simulink model "quadrotorsim_Equations_New_V6B_RC_Only"  (R2019a)
settings: Solver=FixedStepAuto  StartTime=0.0  StopTime=10  FixedStep=1  RelTol=1e-3  EnableMultiTasking=on
undefined symbols (not defined in the file): dev, Main, pwm_output0, px4
libraries: simulink x2, px4lib x1
settings Model: ExtModeTrigDuration=10  Creator=samirbo  LastModifiedBy=MEDELEON
settings SolverCC: PositivePriorityOrder=on
settings DataIOCC: LimitDataPoints=on  SaveFormat=Array  ReturnWorkspaceOutputs=off
settings OptimizationCC: EnhancedBackFolding=on  PassReuseOutputArgsAs=Individual arguments  ExpressionDepthLimit=2147483647  InitFltsAndDblsToZero=on  MaxStackSize=64  OptimizeBlockOrder=speed  DifferentSizesBufferReuse=on  OptimizationCustomize=off
settings DebuggingCC: SaveWithParameterizedLinksMsg=none  UnderspecifiedInitializationDetection=Classic  MergeDetectMultiDrivingBlocksExec=none  SignalResolutionControl=TryResolveAllWithWarning  SolverPrmCheckMsg=warning  MultiTaskDSMMsg=warning  MultiTaskCondExecSysMsg=none  ParameterPrecisionLossMsg=none  ParameterTunabilityLossMsg=error  FcnCallInpInsideContextMsg=warning  StateNameClashWarn=warning  SFUnexpectedBacktrackingDiag=warning  SFNoUnconditionalDefaultTransitionDiag=warning  SFExecutionAtInitializationDiag=none  ArithmeticOperatorsInVariantConditions=warning
settings HardwareCC: ProdBitPerPointer=32  ProdBitPerSizeT=32  ProdBitPerPtrDiffT=32  ProdLargestAtomicInteger=Long  ProdLargestAtomicFloat=Double  ProdWordSize=32  ProdLongLongMode=on  ProdHWDeviceType=ARM Compatible->ARM Cortex
settings ModelReferenceCC: PropagateSignalLabelsOutOfModel=off
settings SFSimCC: SimUseLocalCustomCode=off  MATLABDynamicMemAlloc=off
settings RTWCC: SystemTargetFile=ert.tlc  HardwareBoard=PX4 Pixhawk 2.1 (Cube)  TLCOptions="-aInlineSetEventsForThisBaseRateFcn=TLC_FALSE -aSuppressMultiTaskScheduler=TLC_FALSE  -aRateBasedStepFcn=0"  TemplateMakefile=ert_default_tmf  GenerateReport=on  RTWUseLocalCustomCode=off  Toolchain=GNU Tools for PX4 Autopilots  IncludeHyperlinkInReport=on  LaunchReport=on  TargetLang=C++  GenerateTraceInfo=on  GenerateTraceReport=on  GenerateTraceReportSl=on  GenerateTraceReportSf=on  GenerateTraceReportEml=on  CheckMdlBeforeBuild=Error
settings CodeAppCC: ForceParamTrailComments=on  IgnoreCustomStorageClasses=off  OperatorAnnotations=on  SimulinkDataObjDesc=on  SFDataObjDesc=on  InsertBlockDesc=on
settings ConfigComp: CovMetricSettings=dw  CovHtmlReporting=on  CovSaveCumulativeToWorkspaceVar=on  CovSaveSingleToWorkspaceVar=on  CovExternalEMLEnable=off

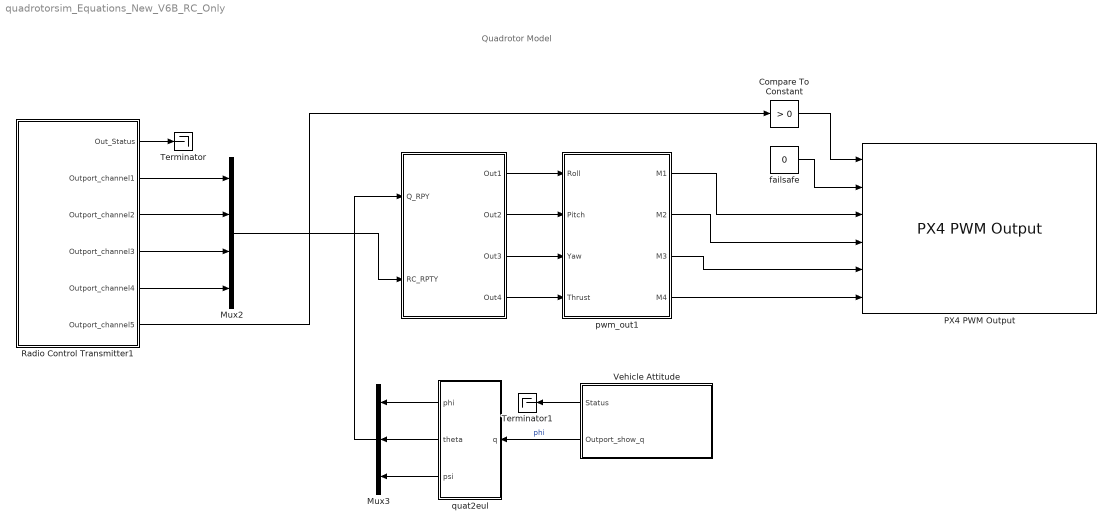
== system quadrotorsim_Equations_New_V6B_RC_Only ==
  note: Quadrotor Model
  " " : Subsystem
      mask Display: disp('Control System')
  Compare To Constant : simulink/Logic and Bit Operations/Compare To Constant  relop=>  const=0  OutDataTypeStr=boolean
  Mux2 : Mux
  Mux3 : Mux  Inputs=3
  PX4 PWM Output : px4lib/PX4 PWM Output  pwmDevice=Main (/dev/pwm_output0)  pwmChannel1_=on  pwmChannel2_=on  pwmChannel3_=on  pwmChannel4_=on  pwmChannel5_=off  pwmChannel6_=off  pwmChannel7_=off  pwmChannel8_=off  forceTerminateFailsafe=off  outputErrorStatus=off
      settings: SourceProductName=Embedded Coder Support Package for PX4 Autopilots  SourceProductBaseCode=PX4AUTOPILOTS
  Radio Control Transmitter1 : Subsystem  AncestorBlock=px4Sensorslib/Radio Control Transmitter  mask(PX4 Radio Control Transmitter){channel1=on, channel2=on, channel3=on, channel4=on, channel5=on, channel6=off, channel7=off, channel8=off, channel_count=off, rssi=off, rc_input_source=off, timestamp_last_signal=off, time_stamp=off, sampleTime=-1, BlockingMode=off, BlockTimeout=5}
      mask prompts: channel1 "px4:blockmask:uORBRCBlockMaskCh1"; channel2 "px4:blockmask:uORBRCBlockMaskCh2"; channel3 "px4:blockmask:uORBRCBlockMaskCh3"; channel4 "px4:blockmask:uORBRCBlockMaskCh4"; channel5 "px4:blockmask:uORBRCBlockMaskCh5"; channel6 "px4:blockmask:uORBRCBlockMaskCh6"; channel7 "px4:blockmask:uORBRCBlockMaskCh7"; channel8 "px4:blockmask:uORBRCBlockMaskCh8"; channel_count "px4:blockmask:uORBRCBlockMaskChCount"; rssi "px4:blockmask:uORBRCBlockMaskRSSI"; rc_input_source "px4:blockmask:uORBRCBlockMaskRCSource"; timestamp_last_signal "px4:blockmask:uORBRCBlockMaskRCTimestampLastSignal"; time_stamp "px4:blockmask:uORBRCBlockMaskTs"; sampleTime "px4:blockmask:SampleTimePrompt"; BlockingMode "px4:blockmask:SubscriberBlockingMode"; BlockTimeout "px4:blockmask:SubscriberBlockingModeTimeout"
      mask help: px4:blockmask:uORBRCBlockMaskDescription
      mask init:
      | signal_names = {'channel_1','channel_2','channel_3','channel_4',...
      |                         'channel_5','channel_6','channel_7','channel_8',...
      |                         '<channel_count>','<rssi>',...
      |                         '<input_source>','<timestamp_last_signal>','<timestamp>'};
      | output_port_names = {'Ch 1','Ch 2','Ch 3',...
      |                         'Ch 4','Ch 5','Ch 6','Ch 7',...
      |                         'Ch 8','Num Ch','RSSI',...
      |                         'RC Source','Last valid time','Timestamp'...
      |                         };
      | mask_image = 'mask_input_rc.png';                    
      | imfilename = fullfile(codertarget.pixhawk.internal.getSpPkgRootDir, 'resources', mask_image);
      | px4.internal.block.CommonuORBTopicMask.commonMaskCallback(gcb,signal_names,output_port_names,imfilename);
      mask Help: eval('codertarget.internal.helpView(''px4'',''px4librctransmitter'')');
      mask TypeOptions sampleTime: PX4 uORB Read/sampleTime
      mask TypeOptions BlockingMode: PX4 uORB Read/BlockingMode
      mask Callback BlockingMode: px4.internal.block.CommonuORBTopicMask.blockingModeCallback(gcb);
      mask TypeOptions BlockTimeout: PX4 uORB Read/BlockTimeout
      mask DialogControl Container10 Prompt: px4:blockmask:uORBRCBlockMainTab
      mask DialogControl Container14 Prompt: px4:blockmask:uORBRCBlockChSelection
      mask DialogControl Container17 Prompt: px4:blockmask:uORBRCBlockAdditionalOp
      mask DialogControl Container19 Prompt: px4:blockmask:uORBRCBlockAdvancedTab
      mask Display:
      | color('white');
      | plot([100,100,100,100],[100,100,100,100]);
      | plot([0,0,0,0],[0,0,0,0]);
      | image('C:\ProgramData\MATLAB\SupportPackages\R2018b\toolbox\target\supportpackages\px4\resources\mask_input_rc.png','center')
      | color('blue');
      | text(0.25, 0.9, 'PX4', 'horizontalAlignment', 'right');
      | color('black');
      | port_label('output',1,'Status');
      | port_label('output',2,'Ch 1');
      | port_label('output',3,'Ch 2');
      | port_label('output',4,'Ch 3');
      | port_label('output',5,'Ch 4');
      | port_label('output',6,'Ch 5');
  Terminator : Terminator
  Terminator1 : Terminator
  Vehicle Attitude : Subsystem  AncestorBlock=px4Sensorslib/Vehicle Attitude  mask(PX4 Vehicle Attitude){rollRate=off, pitchRate=off, yawRate=off, quaternion=on, uorbTimeStamp=off, BlockingMode=off, BlockTimeout=0.001, sampleTime=-1}
      mask prompts: rollRate "Roll Rate"; pitchRate "Pitch Rate"; yawRate "Yaw Rate"; quaternion "Quaternion (NED)"; uorbTimeStamp "Timestamp"; BlockingMode "px4:blockmask:SubscriberBlockingMode"; BlockTimeout "px4:blockmask:SubscriberBlockingModeTimeout"; sampleTime "px4:blockmask:SampleTimePrompt"
      mask help: px4:blockmask:VehicleAttitueBlockMaskDescription
      mask init:
      | signal_names = {'<rollspeed>','<pitchspeed>','<yawspeed>',...
      |     '<q>','<timestamp>'};
      | output_port_names = {'Roll rate','Pitch rate',...
      |     'Yaw rate','Quaternion','Timestamp'};
      | mask_image = fullfile(codertarget.pixhawk.internal.getSpPkgRootDir,...
      |     'resources','mask_vehicle_attitude.png');
      | 
      | px4.internal.block.CommonuORBTopicMask.commonMaskCallback(gcb,...
      |     signal_names,output_port_names,mask_image);
      mask Help: eval('codertarget.internal.helpView(''px4'' ,''px4libvehicleattitude'')')
      mask TypeOptions BlockingMode: PX4 uORB Read/BlockingMode
      mask Callback BlockingMode: px4.internal.block.CommonuORBTopicMask.blockingModeCallback(gcb);
      mask TypeOptions BlockTimeout: PX4 uORB Read/BlockTimeout
      mask TypeOptions sampleTime: PX4 uORB Read/sampleTime
      mask DialogControl Container6 Prompt: Main
      mask DialogControl Container8 Prompt: Advanced
      mask Display:
      | color('white');
      | plot([100,100,100,100],[100,100,100,100]);
      | plot([0,0,0,0],[0,0,0,0]);
      | image('C:\ProgramData\MATLAB\SupportPackages\R2018b\toolbox\target\supportpackages\px4\resources\mask_vehicle_attitude.png','center')
      | color('blue');
      | text(0.25, 0.9, 'PX4', 'horizontalAlignment', 'right');
      | color('black');
      | port_label('output',1,'Status');
      | port_label('output',2,'Quaternion');
  failsafe : Constant  Value=0  OutDataTypeStr=boolean  SampleTime=-1
  pwm_out1 : MATLAB Function  TreatAsAtomicUnit=on
  quat2eul : MATLAB Function  TreatAsAtomicUnit=on
  wires:
  Radio Control Transmitter1/2(Outport_channel1) -> Mux2/1
  Radio Control Transmitter1/3(Outport_channel2) -> Mux2/2
  Radio Control Transmitter1/4(Outport_channel3) -> Mux2/3
  Radio Control Transmitter1/5(Outport_channel4) -> Mux2/4
  quat2eul/2(theta) -> Mux3/2
  quat2eul/1(phi) -> Mux3/1
  quat2eul/3(psi) -> Mux3/3
  Vehicle Attitude/2(Outport_show_q) -> quat2eul/1(q)  "phi"
  " "/1(Out1) -> pwm_out1/1(Roll)
  " "/2(Out2) -> pwm_out1/2(Pitch)
  " "/3(Out3) -> pwm_out1/3(Yaw)
  " "/4(Out4) -> pwm_out1/4(Thrust)
  pwm_out1/1(M1) -> PX4 PWM Output/3
  pwm_out1/2(M2) -> PX4 PWM Output/4
  pwm_out1/3(M3) -> PX4 PWM Output/5
  pwm_out1/4(M4) -> PX4 PWM Output/6
  Mux3/1 -> " "/1(Q_RPY)
  Mux2/1 -> " "/2(RC_RPTY)
  Radio Control Transmitter1/1(Out_Status) -> Terminator/1
  Vehicle Attitude/1(Status) -> Terminator1/1
  Radio Control Transmitter1/6(Outport_channel5) -> Compare To Constant/1
  failsafe/1 -> PX4 PWM Output/2
  Compare To Constant/1 -> PX4 PWM Output/1

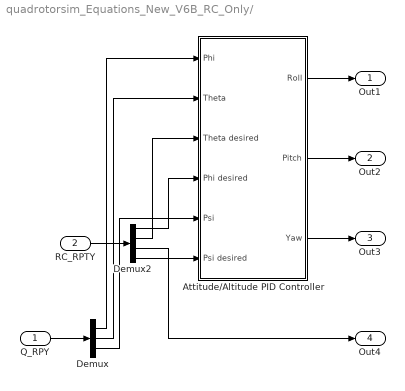
== system quadrotorsim_Equations_New_V6B_RC_Only/  ==
  Q_RPY : Inport
  RC_RPTY : Inport  Port=2
  Attitude/Altitude PID Controller : Subsystem
  Demux : Demux  Outputs=3
  Demux2 : Demux
  Out1 : Outport
  Out2 : Outport  Port=2
  Out3 : Outport  Port=3
  Out4 : Outport  Port=4
  wires:
  Q_RPY/1 -> Demux/1
  Demux/1 -> Attitude/Altitude PID Controller/1(Phi)
  Demux/2 -> Attitude/Altitude PID Controller/2(Theta)
  Demux/3 -> Attitude/Altitude PID Controller/5(Psi)
  RC_RPTY/1 -> Demux2/1
  Attitude/Altitude PID Controller/1(Roll) -> Out1/1
  Attitude/Altitude PID Controller/2(Pitch) -> Out2/1
  Attitude/Altitude PID Controller/3(Yaw) -> Out3/1
  Demux2/1 -> Attitude/Altitude PID Controller/4(Phi desired)
  Demux2/2 -> Attitude/Altitude PID Controller/3(Theta desired)
  Demux2/4 -> Attitude/Altitude PID Controller/6(Psi desired)
  Demux2/3 -> Out4/1

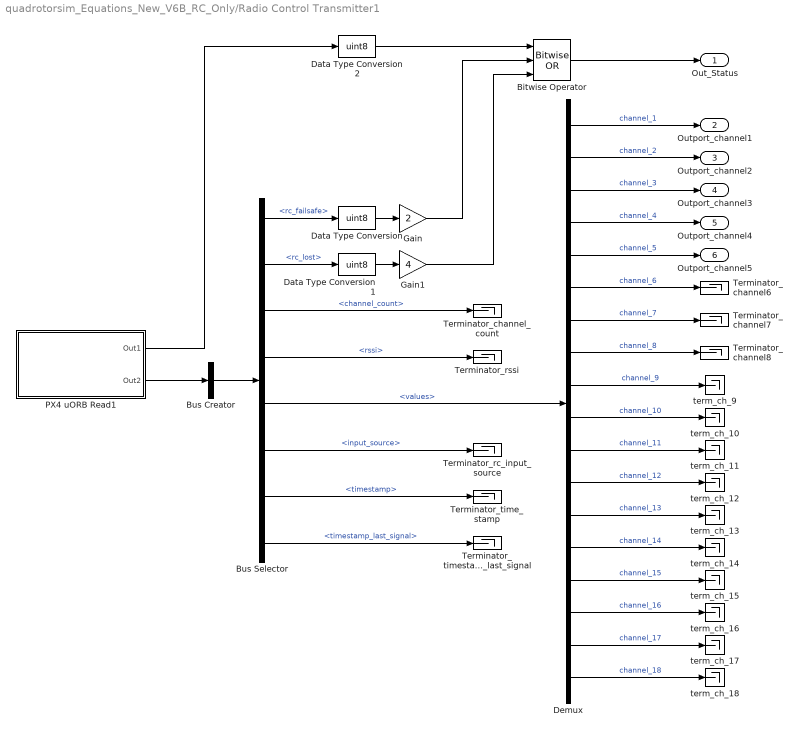
== system quadrotorsim_Equations_New_V6B_RC_Only/Radio Control Transmitter1 ==
  Bitwise Operator : simulink/Logic and Bit Operations/Bitwise Operator  logicop=OR  UseBitMask=off  NumInputPorts=3  BitMask=bin2dec('11011001')  BitMaskRealWorld=Stored Integer
  Bus Creator : BusCreator  Inputs=1
  Bus Selector : BusSelector  OutputSignals=rc_failsafe,rc_lost,channel_count,rssi,values,input_source,timestamp,timestamp_last_signal
  Data Type Conversion : DataTypeConversion  OutDataTypeStr=uint8
  Data Type Conversion1 : DataTypeConversion  OutDataTypeStr=uint8
  Data Type Conversion2 : DataTypeConversion  OutDataTypeStr=uint8
  Demux : Demux  Outputs=18
  Gain : Gain  Gain=2  OutDataTypeStr=uint8
  Gain1 : Gain  Gain=4  OutDataTypeStr=uint8
  PX4 uORB Read1 : Subsystem  AncestorBlock=px4uORBlib/PX4 uORB Read  mask(PX4 uORB Read){uORBTopic=input_rc, sampleTime=-1, BlockingMode=off, BlockTimeout=1e-3}
      mask prompts: uORBTopic "px4:blockmask:TopicPrompt"; sampleTime "px4:blockmask:SampleTimePrompt"; BlockingMode "px4:blockmask:SubscriberBlockingMode"; BlockTimeout "px4:blockmask:SubscriberBlockingModeTimeout"
      mask help: px4:blockmask:SubscriberBlockMaskDescription
      mask init:
      | px4.internal.block.SubscribeBlockMask.dispatch('maskInitialize', gcb);
      settings: ModelCloseFcn=px4.internal.block.SubscribeBlockMask.dispatch('modelCloseFcn', gcb);
      mask Help: eval('codertarget.internal.helpView(''px4'',''px4libuorbread'')');
      mask TypeOptions uORBTopic: SourceBlock/uORBTopic
      mask Callback uORBTopic: px4.internal.block.SubscribeBlockMask.dispatch('topicEdit', gcb);
      mask TypeOptions sampleTime: SourceBlock/SampleTime
      mask TypeOptions BlockingMode: SourceBlock/BlockingMode
      mask Callback BlockingMode: px4.internal.block.SubscribeBlockMask.dispatch('blockingModeSelect', gcb);
      mask TypeOptions BlockTimeout: SourceBlock/BlockTimeout
      mask DialogControl ContainerMain Prompt: px4:blockmask:MainTabTitle
      mask DialogControl topicSelectButton Prompt: px4:blockmask:SelectPrompt
      mask DialogControl topicSelectButton Callback: px4.internal.block.SubscribeBlockMask.dispatch('topicSelect', gcb);
      mask DialogControl ContainerAdvanced Prompt: px4:blockmask:AdvancedTabTitle
      mask Display:
      | color('blue');
      | text(0.2, 0.90, 'PX4', 'horizontalAlignment', 'right');
      | color('black');
      | text(0.5, 0.60, 'uORB Read', 'horizontalAlignment', 'center');
      | if length(uORBTopic) > 16
      |   text(0.83, 0.15, uORBTopic, 'horizontalAlignment', 'right');
      | else
      |   text(0.5, 0.15, uORBTopic, 'horizontalAlignment', 'center');
      | end
      | port_label('output', 1, 'Status');
      | port_label('output', 2, 'Msg');
  Terminator_channel6 : Terminator
  Terminator_channel7 : Terminator
  Terminator_channel8 : Terminator
  Terminator_channel_count : Terminator
  Terminator_rc_input_source : Terminator
  Terminator_rssi : Terminator
  Terminator_time_stamp : Terminator
  Terminator_timestamp_last_signal : Terminator
  "term_ch_10 " : Terminator
  term_ch_{9,11..18} (9 alike) : Terminator
  Out_Status : Outport
  Outport_channel1 : Outport  Port=2
  Outport_channel2 : Outport  Port=3
  Outport_channel3 : Outport  Port=4
  Outport_channel4 : Outport  Port=5
  Outport_channel5 : Outport  Port=6
  wires:
  Data Type Conversion2/1 -> Bitwise Operator/1
  Gain1/1 -> Bitwise Operator/3
  Gain/1 -> Bitwise Operator/2
  PX4 uORB Read1/1(Out1) -> Data Type Conversion2/1
  Bitwise Operator/1 -> Out_Status/1
  Data Type Conversion1/1 -> Gain1/1
  Data Type Conversion/1 -> Gain/1
  Bus Selector/8 -> Terminator_timestamp_last_signal/1  "<timestamp_last_signal>"
  Demux/11 -> term_ch_11/1  "channel_11"
  Demux/3 -> Outport_channel3/1  "channel_3"
  Demux/16 -> term_ch_16/1  "channel_16"
  Demux/13 -> term_ch_13/1  "channel_13"
  Demux/18 -> term_ch_18/1  "channel_18"
  Demux/15 -> term_ch_15/1  "channel_15"
  Bus Selector/3 -> Terminator_channel_count/1  "<channel_count>"
  Demux/17 -> term_ch_17/1  "channel_17"
  Demux/9 -> term_ch_9/1  "channel_9"
  Bus Selector/5 -> Demux/1  "<values>"
  Bus Selector/6 -> Terminator_rc_input_source/1  "<input_source>"
  Demux/10 -> "term_ch_10 "/1  "channel_10"
  Demux/1 -> Outport_channel1/1  "channel_1"
  Demux/12 -> term_ch_12/1  "channel_12"
  Demux/14 -> term_ch_14/1  "channel_14"
  Demux/6 -> Terminator_channel6/1  "channel_6"
  Demux/5 -> Outport_channel5/1  "channel_5"
  Demux/7 -> Terminator_channel7/1  "channel_7"
  Demux/2 -> Outport_channel2/1  "channel_2"
  Demux/8 -> Terminator_channel8/1  "channel_8"
  Demux/4 -> Outport_channel4/1  "channel_4"
  Bus Selector/4 -> Terminator_rssi/1  "<rssi>"
  Bus Selector/1 -> Data Type Conversion/1  "<rc_failsafe>"
  Bus Selector/2 -> Data Type Conversion1/1  "<rc_lost>"
  Bus Selector/7 -> Terminator_time_stamp/1  "<timestamp>"
  PX4 uORB Read1/2(Out2) -> Bus Creator/1
  Bus Creator/1 -> Bus Selector/1

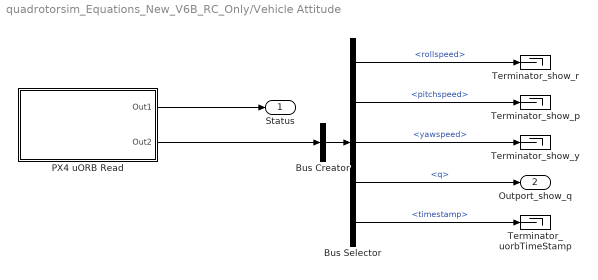
== system quadrotorsim_Equations_New_V6B_RC_Only/Vehicle Attitude ==
  Bus Creator : BusCreator  Inputs=1
  Bus Selector : BusSelector  OutputSignals=rollspeed,pitchspeed,yawspeed,q,timestamp
  PX4 uORB Read : Subsystem  AncestorBlock=px4uORBlib/PX4 uORB Read  mask(PX4 uORB Read){uORBTopic=vehicle_attitude, sampleTime=-1, BlockingMode=off, BlockTimeout=0.001}
      mask prompts: uORBTopic "px4:blockmask:TopicPrompt"; sampleTime "px4:blockmask:SampleTimePrompt"; BlockingMode "px4:blockmask:SubscriberBlockingMode"; BlockTimeout "px4:blockmask:SubscriberBlockingModeTimeout"
      mask help: px4:blockmask:SubscriberBlockMaskDescription
      mask init:
      | px4.internal.block.SubscribeBlockMask.dispatch('maskInitialize', gcb);
      settings: ModelCloseFcn=px4.internal.block.SubscribeBlockMask.dispatch('modelCloseFcn', gcb);
      mask Help: eval('codertarget.internal.helpView(''px4'',''px4libuorbread'')');
      mask TypeOptions uORBTopic: SourceBlock/uORBTopic
      mask Callback uORBTopic: px4.internal.block.SubscribeBlockMask.dispatch('topicEdit', gcb);
      mask TypeOptions sampleTime: SourceBlock/SampleTime
      mask TypeOptions BlockingMode: SourceBlock/BlockingMode
      mask Callback BlockingMode: px4.internal.block.SubscribeBlockMask.dispatch('blockingModeSelect', gcb);
      mask TypeOptions BlockTimeout: SourceBlock/BlockTimeout
      mask DialogControl ContainerMain Prompt: px4:blockmask:MainTabTitle
      mask DialogControl topicSelectButton Prompt: px4:blockmask:SelectPrompt
      mask DialogControl topicSelectButton Callback: px4.internal.block.SubscribeBlockMask.dispatch('topicSelect', gcb);
      mask DialogControl ContainerAdvanced Prompt: px4:blockmask:AdvancedTabTitle
      mask Display:
      | color('blue');
      | text(0.2, 0.90, 'PX4', 'horizontalAlignment', 'right');
      | color('black');
      | text(0.5, 0.60, 'uORB Read', 'horizontalAlignment', 'center');
      | if length(uORBTopic) > 16
      |   text(0.83, 0.15, uORBTopic, 'horizontalAlignment', 'right');
      | else
      |   text(0.5, 0.15, uORBTopic, 'horizontalAlignment', 'center');
      | end
      | port_label('output', 1, 'Status');
      | port_label('output', 2, 'Msg');
  Terminator_show_p : Terminator
  Terminator_show_r : Terminator
  Terminator_show_y : Terminator
  Terminator_uorbTimeStamp : Terminator
  Status : Outport
  Outport_show_q : Outport  Port=2
  wires:
  Bus Selector/5 -> Terminator_uorbTimeStamp/1  "<timestamp>"
  Bus Selector/4 -> Outport_show_q/1  "<q>"
  Bus Selector/1 -> Terminator_show_r/1  "<rollspeed>"
  PX4 uORB Read/1(Out1) -> Status/1
  Bus Selector/2 -> Terminator_show_p/1  "<pitchspeed>"
  Bus Selector/3 -> Terminator_show_y/1  "<yawspeed>"
  PX4 uORB Read/2(Out2) -> Bus Creator/1
  Bus Creator/1 -> Bus Selector/1

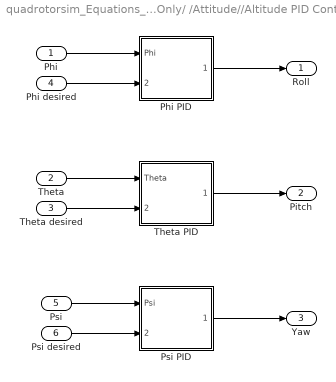
== system quadrotorsim_Equations_New_V6B_RC_Only/ /Attitude//Altitude PID Controller ==
  Phi : Inport
  Theta : Inport  Port=2
  Theta desired : Inport  Port=3
  Phi desired : Inport  Port=4
  Psi : Inport  Port=5
  Psi desired : Inport  Port=6
  Phi PID : Subsystem
  Psi PID : Subsystem
  Theta PID : Subsystem
  Roll : Outport
  Pitch : Outport  Port=2
  Yaw : Outport  Port=3
  wires:
  Phi desired/1 -> Phi PID/2(Phi desired)
  Phi/1 -> Phi PID/1(Phi)
  Psi desired/1 -> Psi PID/2(Psi desired)
  Psi/1 -> Psi PID/1(Psi)
  Theta desired/1 -> Theta PID/2(Theta desired)
  Theta/1 -> Theta PID/1(Theta)
  Phi PID/1(p desired) -> Roll/1
  Psi PID/1(r desired) -> Yaw/1
  Theta PID/1(q desired) -> Pitch/1

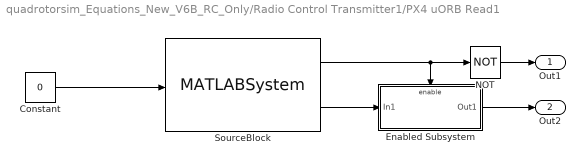
== system quadrotorsim_Equations_New_V6B_RC_Only/Radio Control Transmitter1/PX4 uORB Read1 ==
  Constant : Constant  Value=0  SampleTime=-1
  Enabled Subsystem : Subsystem  TreatAsAtomicUnit=on
  NOT : Logic  Operator=NOT  IconShape=distinctive  AllPortsSameDT=off  OutDataTypeStr=boolean
  SourceBlock : MATLABSystem  InitFcn=px4.internal.block.SubscribeBlockMask.dispatch('sysobjInitFcn', gcb);  System=px4.internal.block.Subscriber  uORBTopic=input_rc  SLBusName=px4_Bus_input_rc  SampleTime=-1  BlockingMode=off  BlockTimeout=1e-3
      mask Type: px4.internal.block.Subscriber
      mask Display:
      | disp('Subscriber');
      | port_label('input',1,'busstruct');
      | port_label('output',1,'isNewData');
      | port_label('output',2,'msg');
  Out1 : Outport
  Out2 : Outport  Port=2
  wires:
  NOT/1 -> Out1/1
  Enabled Subsystem/1(Out1) -> Out2/1
  SourceBlock/1 -> NOT/1, Enabled Subsystem/Enable
  SourceBlock/2 -> Enabled Subsystem/1(In1)
  Constant/1 -> SourceBlock/1

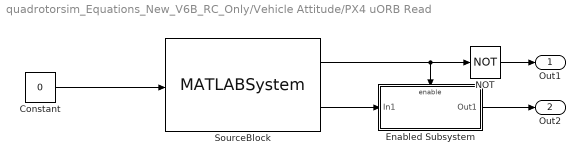
== system quadrotorsim_Equations_New_V6B_RC_Only/Vehicle Attitude/PX4 uORB Read ==
  Constant : Constant  Value=0  SampleTime=-1
  Enabled Subsystem : Subsystem  TreatAsAtomicUnit=on
  NOT : Logic  Operator=NOT  IconShape=distinctive  AllPortsSameDT=off  OutDataTypeStr=boolean
  SourceBlock : MATLABSystem  InitFcn=px4.internal.block.SubscribeBlockMask.dispatch('sysobjInitFcn', gcb);  System=px4.internal.block.Subscriber  uORBTopic=vehicle_attitude  SLBusName=px4_Bus_vehicle_attitude  SampleTime=-1  BlockingMode=off  BlockTimeout=0.001
      mask Type: px4.internal.block.Subscriber
      mask Display:
      | disp('Subscriber');
      | port_label('input',1,'busstruct');
      | port_label('output',1,'isNewData');
      | port_label('output',2,'msg');
  Out1 : Outport
  Out2 : Outport  Port=2
  wires:
  NOT/1 -> Out1/1
  Enabled Subsystem/1(Out1) -> Out2/1
  SourceBlock/1 -> NOT/1, Enabled Subsystem/Enable
  SourceBlock/2 -> Enabled Subsystem/1(In1)
  Constant/1 -> SourceBlock/1

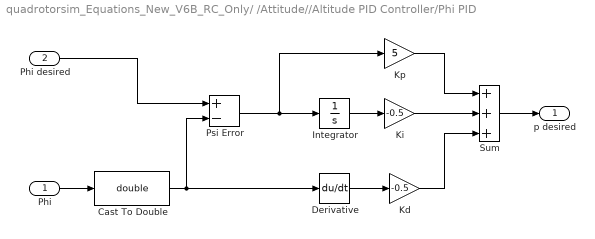
== system quadrotorsim_Equations_New_V6B_RC_Only/ /Attitude//Altitude PID Controller/Phi PID ==
  Phi : Inport
  Phi desired : Inport  Port=2
  Cast To Double : DataTypeConversion  OutDataTypeStr=double
  Derivative : Derivative
  Integrator : Integrator
  Kd : Gain  Gain=-0.5
  Ki : Gain  Gain=-0.5
  Kp : Gain  Gain=5
  Psi Error : Sum  Inputs=+-
  Sum : Sum  Inputs=+++
  p desired : Outport
  wires:
  Phi desired/1 -> Psi Error/1
  Derivative/1 -> Kd/1
  Kp/1 -> Sum/1
  Sum/1 -> p desired/1
  Psi Error/1 -> Integrator/1, Kp/1
  Integrator/1 -> Ki/1
  Kd/1 -> Sum/3
  Ki/1 -> Sum/2
  Phi/1 -> Cast To Double/1
  Cast To Double/1 -> Psi Error/2, Derivative/1

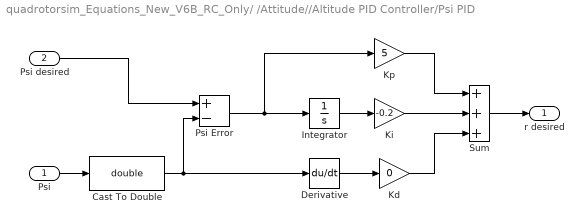
== system quadrotorsim_Equations_New_V6B_RC_Only/ /Attitude//Altitude PID Controller/Psi PID ==
  Psi : Inport
  Psi desired : Inport  Port=2
  Cast To Double : DataTypeConversion  OutDataTypeStr=double
  Derivative : Derivative
  Integrator : Integrator
  Kd : Gain  Gain=0
  Ki : Gain  Gain=-0.2
  Kp : Gain  Gain=5
  Psi Error : Sum  Inputs=+-
  Sum : Sum  Inputs=+++
  r desired : Outport
  wires:
  Psi desired/1 -> Psi Error/1
  Derivative/1 -> Kd/1
  Kp/1 -> Sum/1
  Sum/1 -> r desired/1
  Psi Error/1 -> Integrator/1, Kp/1
  Integrator/1 -> Ki/1
  Kd/1 -> Sum/3
  Ki/1 -> Sum/2
  Psi/1 -> Cast To Double/1
  Cast To Double/1 -> Psi Error/2, Derivative/1

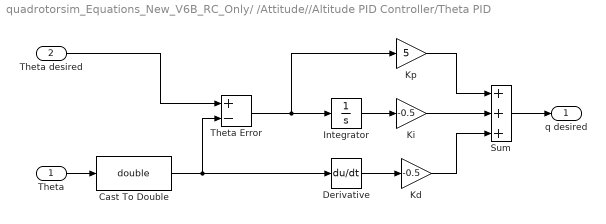
== system quadrotorsim_Equations_New_V6B_RC_Only/ /Attitude//Altitude PID Controller/Theta PID ==
  Theta : Inport
  Theta desired : Inport  Port=2
  Cast To Double : DataTypeConversion  OutDataTypeStr=double
  Derivative : Derivative
  Integrator : Integrator
  Kd : Gain  Gain=-0.5
  Ki : Gain  Gain=-0.5
  Kp : Gain  Gain=5
  Sum : Sum  Inputs=+++
  Theta Error : Sum  Inputs=+-
  q desired : Outport
  wires:
  Theta desired/1 -> Theta Error/1
  Derivative/1 -> Kd/1
  Kp/1 -> Sum/1
  Sum/1 -> q desired/1
  Theta Error/1 -> Integrator/1, Kp/1
  Integrator/1 -> Ki/1
  Kd/1 -> Sum/3
  Ki/1 -> Sum/2
  Theta/1 -> Cast To Double/1
  Cast To Double/1 -> Derivative/1, Theta Error/2

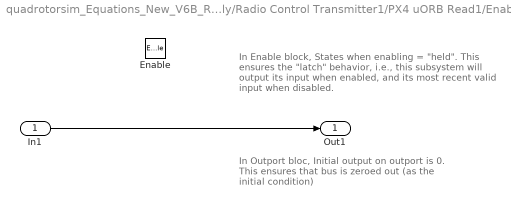
== system quadrotorsim_Equations_New_V6B_RC_Only/Radio Control Transmitter1/PX4 uORB Read1/Enabled Subsystem ==
  note: In Outport bloc, Initial output on outport is 0.
      | This ensures that bus is zeroed out
      | (as the initial condition)
  note: In Enable block, States when enabling = "held".
      | This ensures the "latch" behavior, i.e., this subsystem
      | will output its input when enabled, and its most recent
      | valid input when disabled.
  In1 : Inport
  Enable : EnablePort
  Out1 : Outport  InitialOutput=0
  wires:
  In1/1 -> Out1/1

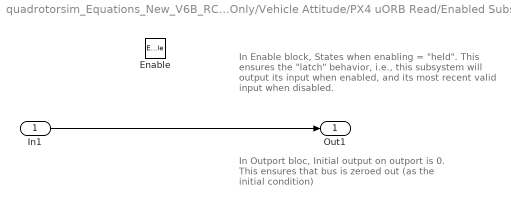
== system quadrotorsim_Equations_New_V6B_RC_Only/Vehicle Attitude/PX4 uORB Read/Enabled Subsystem ==
  note: In Outport bloc, Initial output on outport is 0.
      | This ensures that bus is zeroed out
      | (as the initial condition)
  note: In Enable block, States when enabling = "held".
      | This ensures the "latch" behavior, i.e., this subsystem
      | will output its input when enabled, and its most recent
      | valid input when disabled.
  In1 : Inport
  Enable : EnablePort
  Out1 : Outport  InitialOutput=0
  wires:
  In1/1 -> Out1/1

== matlab function quadrotorsim_Equations_New_V6B_RC_Only/pwm_out1 ==
  data: Roll input; M1 output; Pitch input; Yaw input; Thrust input; M2 output; M3 output; M4 output
function [M1, M2, M3, M4] = motor_mixer(Roll, Pitch, Yaw, Thrust)


idle_PWM = uint16(1000);


% Quad X
M1 = ((Roll + Pitch - Yaw) / 2 * Thrust + Thrust) * 1000 + idle_PWM;
M2 = ((-Roll + Pitch + Yaw) / 2 * Thrust + Thrust) * 1000 + idle_PWM;
M3 = ((-Roll - Pitch - Yaw) / 2 * Thrust + Thrust) * 1000 + idle_PWM;
M4 = ((Roll - Pitch + Yaw) / 2 * Thrust + Thrust) * 1000 + idle_PWM;
% M5 = 1000;
% M6 = 1000;
% M7 = 1000;
% M8 = 1000;

% Quad +
% M1 = ((Pitch - Yaw) * Thrust / 2 + Thrust) * 1000 + idle_PWM;
% M2 = ((-Roll + Yaw) * Thrust / 2 + Thrust) * 1000 + idle_PWM;
% M3 = ((-Pitch - Yaw) * Thrust / 2 + Thrust) * 1000 + idle_PWM;
% M4 = ((Roll + Yaw) * Thrust / 2 + Thrust) * 1000 + idle_PWM;
% M5 = 1000;
% M6 = 1000;
% M7 = 1000;
% M8 = 1000;

% Hex X
% M1 = ((Pitch + Roll / 2 - Yaw) * Thrust / 2 + Thrust) * 1000 + idle_PWM;
% M2 = ((Pitch - Roll / 2 + Yaw) * Thrust / 2 + Thrust) * 1000 + idle_PWM;
% M3 = ((-Roll - Yaw) * Thrust / 2 + Thrust) * 1000 + idle_PWM;
% M4 = ((-Pitch - Roll / 2 + Yaw) * Thrust / 2 + Thrust) * 1000 + idle_PWM;
% M5 = ((-Pitch + Roll / 2 - Yaw) * Thrust / 2 + Thrust) * 1000 + idle_PWM;
% M6 = ((Roll + Yaw) * Thrust / 2 + Thrust) * 1000 + idle_PWM;
% M7 = 1000;
% M8 = 1000;

% Hex X (From Adam)
%M1 = uint16(single(((-Roll - Yaw) * Thrust / 3 + Thrust) * single(1000))) + idle_PWM;
%M2 = uint16(single(((Roll + Yaw) * Thrust / 3 + Thrust) * single(1000))) + idle_PWM;
%M3 = uint16(single(((Pitch + (Roll / 2) - Yaw) * Thrust / 3 + Thrust) * single(1000))) + idle_PWM;
%M4 = uint16(single(((-Pitch - (Roll / 2) + Yaw) * Thrust / 3 + Thrust) * single(1000))) + idle_PWM;
%M5 = uint16(single(((Pitch - (Roll / 2) + Yaw) * Thrust / 3 + Thrust) * single(1000))) + idle_PWM;
%M6 = uint16(single(((-Pitch + (Roll / 2) - Yaw) * Thrust / 3 + Thrust) * single(1000))) + idle_PWM;

% Hex X (Version 2)
% Roll/Yaw
% M1 = ((-Roll - Yaw) * Thrust / 2 + Thrust) * 1000 + idle_PWM;
% M2 = ((Roll + Yaw) * Thrust / 2 + Thrust) * 1000 + idle_PWM;
% % + Pitch/Roll
% M6 = ((Pitch + Roll / 2 - Yaw) * Thrust / 2 + Thrust) * 1000 + idle_PWM;
% M4 = ((Pitch - Roll / 2 + Yaw) * Thrust / 2 + Thrust) * 1000 + idle_PWM;
% % - Pitch/Roll
% M5 = ((-Pitch - Roll / 2 + Yaw) * Thrust / 2 + Thrust) * 1000 + idle_PWM;
% M3 = ((-Pitch + Roll / 2 - Yaw) * Thrust / 2 + Thrust) * 1000 + idle_PWM;

== matlab function quadrotorsim_Equations_New_V6B_RC_Only/quat2eul ==
  data: q input; phi output; theta output; psi output
function [phi,theta,psi] = quat2eul(q)
% Conversion from Quaternion to Euler angles based on the PX4 Firmware
% v1.6.5 release.
% 
% Quaternion -> DCM -> Euler Angles
% INPUT:
%   q: Quaternion vector of the format: (a + bi + cj + dk)
% OUTPUT:
%   [phi,theta,psi]: Euler angles in radians.
% 
 
    a = q(1);
    b = q(2);
    c = q(3);
    d = q(4);

    aSq = a*a;
    bSq = b*b;
    cSq = c*c;
    dSq = d*d;

    d_pi2 = pi/2;

    % quaternion_to_dcm
    dcm00 = aSq + bSq - cSq - dSq;
    % dcm01 = 2*(b*c - a*d);
    dcm02 = 2*(a*c + b*d);
    dcm10 = 2*(b*c + a*d);
    % dcm11 = aSq - bSq + cSq - dSq;
    dcm12 = 2*(c*d - a*b);
    dcm20 = 2*(b*d - a*c);
    dcm21 = 2*(a*b + c*d);
    dcm22 = aSq - bSq - cSq + dSq;

    % dcm_to_euler
    theta = asin(-dcm20);
    if abs(theta - d_pi2) < 1.0e-3
        phi = single(0.0);
        psi = atan2(dcm12, dcm02);
    elseif abs(theta + d_pi2) < 1.0e-3
        phi = single(0.0);
        psi = atan2(-dcm12, -dcm02);
    else
        phi = atan2(dcm21, dcm22);
        psi = atan2(dcm10, dcm00);
    end

end
